simulink model "sar12"  (R2022b)
settings: Solver=VariableStepAuto  StartTime=0.0  StopTime=16.5e-3  RelTol=1e-3
InitFcn:
  | rng('default');
  | 
  | SampCap = 2^11*2*50e-15;
  | 
  | Npoints = 8192;
  | 
  | fs=500000;
  | 
  | %fin=743*fs/Npoints;
  | fin=419*fs/Npoints;
  | 
  | 
  | 
  | Comp_os = 0;
  | 
  | Cu = 50e-15;
  | del_Cu = 0.01*Cu;
  | Wda = [2048; 1024; 512; 256; 128; 64; 32; 16; 8; 4; 2; 1;];
  | 
  | for i=1:12
  | 
  |     rng('shuffle');  % 根据当前时间和其他状态设置随机种子
  |     Cm_p(i) = Wda(i)*Cu+sqrt(Wda(i))*del_Cu*randn(1,1);
  | 
  |     rng('shuffle');  % 根据当前时间和其他状态设置随机种子
  |     Cm_n(i) = Wda(i)*Cu+sqrt(Wda(i))*del_Cu*randn(1,1);
  | 
  | end
  | 
  | rng('shuffle');  % 根据当前时间和其他状态设置随机种子
  | Cd_p = 1*Cu+sqrt(1)*del_Cu*randn(1,1);
  | 
  | rng('shuffle');  % 根据当前时间和其他状态设置随机种子
  | Cd_n = 1*Cu+sqrt(1)*del_Cu*randn(1,1);
undefined symbols (not defined in the file or in its folder): clock, Cm_n, Cm_p
libraries: SDtoolbox x7
settings Model: Creator=R5  LastModifiedBy=DELL
settings OptimizationCC: ReuseModelBlockBuffer=on

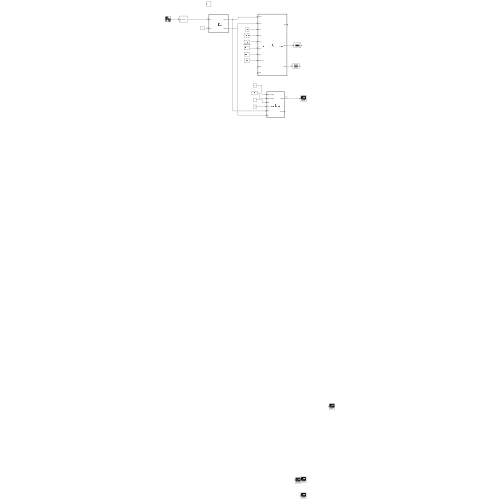
[thumbnail: Simulink's stored preview of the top-level diagram]
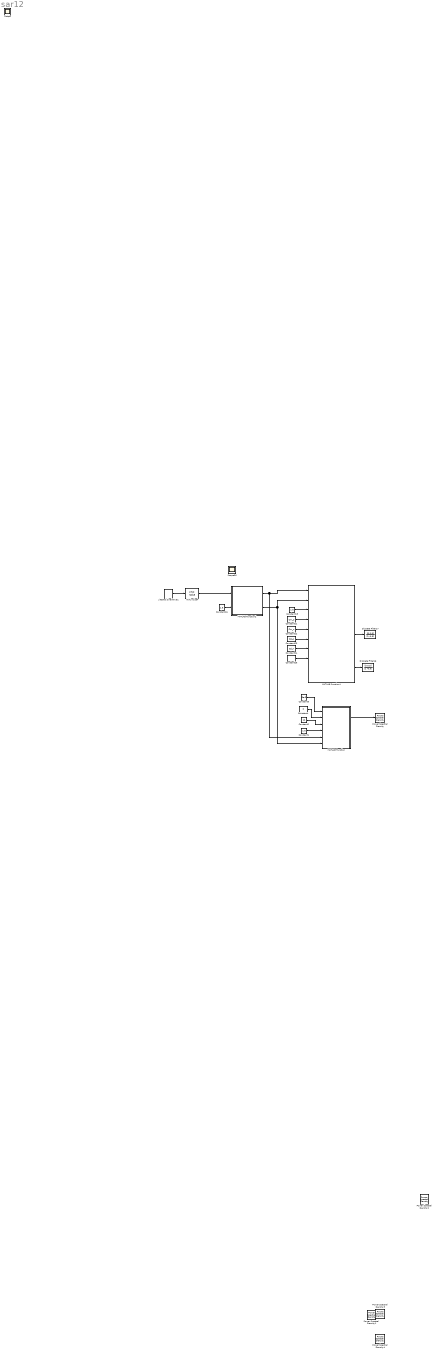
== system sar12 ==
  Constant1 : Constant  Value=1.6
  Constant16 : Constant  Value=1.6
  Constant19 : Constant  Value=1.6
  Constant2 : Constant  Value=12
  Constant21 : Constant  Value=Cm_p
  Constant22 : Constant  Value=Cm_n
  Constant23 : Constant  Value=Cd_p
  Constant24 : Constant  Value=Cd_n
  Constant26 : Constant  Value=Comp_os
  Constant3 : Constant  Value=5e-3
  Constant4 : Constant  Value=0
  Discrete Filter16 : DiscreteFilter  Numerator=[0 0.5]  Denominator=[1 -0.5]
  Discrete Filter17 : DiscreteFilter  Numerator=[0 0.5]  Denominator=[1 -0.5]
  Jittered SineWave1 : SDtoolbox/Jittered SineWave  Ampl=1.5  Bias=0  Freq=fin*2*pi  Phase=0  SampJ=0  Ts=1/fs  seed=1
      settings: SourceProductName=SDtoolbox
  MATLAB Function : MATLAB Function  TreatAsAtomicUnit=on
  MATLAB Function2 : MATLAB Function  TreatAsAtomicUnit=on
  MATLAB Function4 : MATLAB Function  TreatAsAtomicUnit=on
  Power Spectral Density : SDtoolbox/Power Spectral Density  SN=2  Fs=fs  fBL=fs/Npoints*3  fBH=fs/2  Fin=fin  N=Npoints  Ntransient=10  VW=off  savename=savemat  Scale_type=logarithmic
      settings: SourceProductName=SDtoolbox
  Power Spectral Density{1..4} (4 alike) : SDtoolbox/Power Spectral Density  SN=1  Fs=fs  fBL=fs/Npoints*3  fBH=125000  Fin=fin  N=Npoints  Ntransient=10  VW=on  savename=savemat  Scale_type=logarithmic
      settings: SourceProductName=SDtoolbox
  Scope36 : Scope
  kT/C noise4 : SDtoolbox/kT//C noise  Ts=1/fs  C=SampCap  Temp=300  k=1.38e-23  seed=floor(sum(2.6451561*clock))
      settings: SourceProductName=SDtoolbox
  Scope : Scope
  wires:
  Constant21/1 -> MATLAB Function4/4(Cm_p)
  Constant24/1 -> MATLAB Function4/7(Cd_n)
  Jittered SineWave1/1 -> kT/C noise4/1
  MATLAB Function2/1(OUT1P) -> MATLAB Function/5(vip), MATLAB Function4/1(Vin1p)
  Constant23/1 -> MATLAB Function4/6(Cd_p)
  Constant16/1 -> MATLAB Function2/2(Vref)
  Constant19/1 -> MATLAB Function4/3(Vref)
  MATLAB Function2/2(OUT1N) -> MATLAB Function/6(vin), MATLAB Function4/2(Vin1n)
  MATLAB Function4/2(Vresp) -> Discrete Filter17/1
  MATLAB Function4/3(Vresn) -> Discrete Filter16/1
  Constant22/1 -> MATLAB Function4/5(Cm_n)
  Constant26/1 -> MATLAB Function4/8(Comp_os)
  kT/C noise4/1 -> MATLAB Function2/1(IN1)
  Constant1/1 -> MATLAB Function/4(vref)
  Constant2/1 -> MATLAB Function/3(nbit)
  Constant3/1 -> MATLAB Function/1(del_Compos)
  Constant4/1 -> MATLAB Function/2(del_Compvn)
  MATLAB Function/1(outAD) -> Power Spectral Density/1

== matlab function sar12/MATLAB Function ==
  data: outAD output; del_Compos input; D1out output; del_Compvn input; nbit input; vref input; vip input; vin input
function [outAD,D1out] =binary_ADCnbit(del_Compos,del_Compvn,nbit,vref,vip,vin)

%nbit SAR ADC%
N=nbit+1;  %10bit需要11个电容
outAD=0;
dout=zeros(nbit,1);
D1out=zeros(100,1);
C_nor=zeros(1,N);
Comp_os=del_Compos*randn(1,1);
% D2out=zeros(7,1);

Vos2=0;%失调电压

%------Mismatch Parameter------%

C_nor(1)=1;
for i=N:-1:2
    C_nor(i)=2^(i-2);
end
%C_nor = [1 1 2 4 8 16 32 64 128 256 512 1024 2048]; %
C=[C_nor C_nor];
sig_c = 0.0; % 定义单位电容的标准偏差，其值为0，故电容失配此时为0.
rng(10,'twister');% 指定种子数，twister是生成器,randn的标志，保证每次运行时生成
C_dev = sig_c*sqrt(C).*randn(1,2*(N)); % 每次运算具有不同的失配误差
C_devp=C_dev(1:N);
C_devn=C_dev(N+1:2*N);%前n位给p端电容，后n位给n端电容

%------DAC array------%

capp = C_nor' + C_devp'; % 定义实际电容由其均值和标准偏差组成
capn = C_nor' + C_devn';
captotp=sum(capp);      %total cap
captotn=sum(capn);      %total cap

%Converting%逐次逼近的过程，哪个数大后面就是加号，反之就是减号
if ((vip+Vos2+Comp_os+del_Compvn*randn(1,1)) < (vin))
       vip=vip+(vref/2)*(capp(N)/(captotp));
       vin=vin-(vref/2)*(capn(N)/(captotn));
       dout(nbit)=0;
       D1out(1)=0;

 else
       vip=vip-(vref/2)*(capp(N)/(captotp));
       vin=vin+(vref/2)*(capn(N)/(captotn));
       dout(nbit)=1;
       D1out(1)=1;
end


for k=(nbit-1):-1:1
    if ((vip+Vos2+Comp_os+del_Compvn*randn(1,1)) < (vin))
       vip=vip+(vref/2)*(capp(k+1)/(captotp));
       vin=vin-(vref/2)*(capn(k+1)/(captotn));
       dout(k)=0;
       D1out(N-k)=0;
    else
       vip=vip-(vref/2)*(capp(k+1)/(captotp));
       vin=vin+(vref/2)*(capn(k+1)/(captotn));
       dout(k)=1;
       D1out(N-k)=1;
    end
end
for k=(nbit):-1:1
    outAD=outAD+D1out(k)*2^(nbit-k);
end

end

== matlab function sar12/MATLAB Function2 ==
  data: IN1 input; OUT1P output; Vref input; OUT1N output
function [OUT1P, OUT1N] = Single2Dual(IN1, Vref)
    Vcm = Vref/2;
    OUT1P = Vcm + 0.5*IN1;
    OUT1N = Vcm - 0.5*IN1;
end

== matlab function sar12/MATLAB Function4 ==
  data: Dout output; Vin1p input; Vin1n input; Vresp output; Vref input; Cm_p input; Cm_n input; Cd_p input; Cd_n input; Comp_os input; Vintp input; Vintn input; Vresn output
function [Dout, Vresp, Vresn] = VCM_based_SAR_and_ADDER(Vin1p, Vin1n, Vref, Cm_p, Cm_n, Cd_p, Cd_n, Comp_os, Vintp, Vintn)
Vcm = Vref/2;
M = 12;
Vdamp = Vcm * ones(1,M);
Vdamn = Vcm * ones(1,M);
Wda = [2048 1024 512 256 128 64 32 16 8 4 2 1];
Ctot_p = sum(Cm_p) + Cd_p;
Ctot_n = sum(Cm_n) + Cd_n;
Qp = (Vin1p-Vcm) * Ctot_p;
Qn = (Vin1n-Vcm) * Ctot_n;

for i = 1:M
    Vresp = (Qp + Vcm*Cd_p + Vdamp*Cm_p)/Ctot_p ;
    Vresn = (Qn + Vcm*Cd_n + Vdamn*Cm_n)/Ctot_n ;

    if Vresp + Vintp + Comp_os > Vresn + Vintn
        Vdamp(i) = 0;
        Vdamn(i) = Vref;
    else
        Vdamp(i) = Vref;
        Vdamn(i) = 0;
        Wda(i) = 0;
    end

end

    Vresp = (Qp + Vcm*Cd_p + Vdamp*Cm_p)/Ctot_p ;
    Vresn = (Qn + Vcm*Cd_n + Vdamn*Cm_n)/Ctot_n ;


Dout = sum(Wda);

end
